simulink library "mylib"  (Simulink 9.2)
settings: Solver=VariableStepAuto  StartTime=0.0  StopTime=10.0  RelTol=1e-3
values from neighbouring files (symbols this model uses):
  FLINT32_MAX = flintmax('single')    [lib_consts.m]
undefined symbols (not defined in the file or in its folder): BAR_2_Pa, CC_2_M3, CCpREV_2_M3pRAD, DEG_2_RAD, DiscIntNeverNeededParam, G_2_MPS2, KNOTS_2_KPH, KPH_2_KNOTS, KPH_2_MPS, kXX_2_XX, M3_2_CC, M3pRAD_2_CCpREV, MPS2_2_G, MPS_2_KPH, Pa_2_BAR, RAD_2_DEG, RADpS_2_RPM, RPM_2_RADpS, XX_2_kXX
libraries: $bdroot x12, simulink x4, Ricardo_SW_dev_lib x1
(part 2 of 2)

== system mylib/Universals/Subsystem ==
  In1 : Inport
      settings: AttributesFormatString=<tsample=%<SampleTime>>
  Out1 : Outport
      settings: AttributesFormatString=<tsample=%<SampleTime>>
  wires:
  In1/1 -> Out1/1

== system mylib/Universals/Switch Case Action Subsystem ==
  In1 : Inport
      settings: AttributesFormatString=<tsample=%<SampleTime>>
  Action Port : ActionPort  ActionType=case
  Out1 : Outport
      settings: AttributesFormatString=<tsample=%<SampleTime>>
  wires:
  In1/1 -> Out1/1

== system mylib/Universals/Variant Subsystem ==
  note: 1) Only subsystems can be added as variant choices at this level
      | 2) Blocks cannot be connected at this level as connectivity is
      | automatically determined at simulation, based on the active variant
  In1 : Inport
      settings: AttributesFormatString=<tsample=%<SampleTime>>
  Out1 : Outport
      settings: AttributesFormatString=<tsample=%<SampleTime>>

== system mylib/Counter&Timer/Counter_Up/Delay_IV ==
  u : Inport
  IV : Inport  Port=2
  Constant4 : Constant  Value=0
  Data Type Conversion4 : DataTypeConversion
  Switch : Switch  Criteria=u2 ~= 0  Threshold=0.5  RndMeth=Zero
      settings: AttributesFormatString=<threshold=%<threshold>>\n<criteria=%<Criteria>>
  Unit Delay : UnitDelay  InitialCondition=1  SampleTime=-1
      settings: AttributesFormatString=<initial=%<x0>>\n<tsample=%<sampleTime>>
  Unit Delay1 : UnitDelay  SampleTime=-1
      settings: AttributesFormatString=<initial=%<x0>>\n<tsample=%<sampleTime>>
  y : Outport
  wires:
  Data Type Conversion4/1 -> Unit Delay/1
  Constant4/1 -> Data Type Conversion4/1
  IV/1 -> Switch/1
  u/1 -> Unit Delay1/1
  Switch/1 -> y/1
  Unit Delay/1 -> Switch/2
  Unit Delay1/1 -> Switch/3

== system mylib/Counter&Timer/rolling_edge_counter/boolean_edge ==
  note: Detect false to true boolean edge
  input_flg : Inport
      settings: AttributesFormatString=<tsample=%<SampleTime>>
  Logical Operator1 : Logic  AllPortsSameDT=off  OutDataTypeStr=boolean
  Logical Operator2 : Logic  Operator=NOT  AllPortsSameDT=off  OutDataTypeStr=boolean
  Unit Delay : UnitDelay  InitialCondition=false  SampleTime=-1
      settings: AttributesFormatString=<initial=%<x0>>\n<tsample=%<sampleTime>>
  edgle_flg : Outport
      settings: AttributesFormatString=<tsample=%<SampleTime>>
  wires:
  Unit Delay/1 -> Logical Operator2/1
  Logical Operator2/1 -> Logical Operator1/2
  Logical Operator1/1 -> edgle_flg/1  "edgle_flg"
  input_flg/1 -> Unit Delay/1, Logical Operator1/1  "input_flg"

== system mylib/Counter&Timer/rolling_edge_counter/conditional_counter ==
  note: Increment a rolling counter each time an edge is detected
  increment_on : Inport
      settings: AttributesFormatString=<tsample=%<SampleTime>>
  Constant : Constant  OutDataTypeStr=uint8  SampleTime=-1
      settings: AttributesFormatString=<tsample=%<SampleTime>>
  Sum : Sum  AccumDataTypeStr=uint8  RndMeth=Zero
  Switch : Switch  Criteria=u2 ~= 0  Threshold=0.5  RndMeth=Zero
      settings: AttributesFormatString=<threshold=%<threshold>>\n<criteria=%<Criteria>>
  Unit Delay1 : UnitDelay  SampleTime=-1
      settings: AttributesFormatString=<initial=%<x0>>\n<tsample=%<sampleTime>>
  rolling_ctr : Outport
      settings: AttributesFormatString=<tsample=%<SampleTime>>
  wires:
  increment_on/1 -> Switch/2  "increment_on"
  Constant/1 -> Sum/1
  Unit Delay1/1 -> Switch/3, Sum/2
  Sum/1 -> Switch/1
  Switch/1 -> Unit Delay1/1, rolling_ctr/1  "rolling_ctr"

== system mylib/PIDs/PI_FeedForward/clip_status ==
  max_dmd : Inport
      settings: AttributesFormatString=<tsample=%<SampleTime>>
  value : Inport  Port=2
      settings: AttributesFormatString=<tsample=%<SampleTime>>
  min_dmd : Inport  Port=3
      settings: AttributesFormatString=<tsample=%<SampleTime>>
  AboveMax : RelationalOperator  Operator=<  OutDataTypeStr=boolean  RndMeth=Nearest
  BelowMin : RelationalOperator  Operator=<  OutDataTypeStr=boolean  RndMeth=Nearest
  OutsideLimit : Logic  Operator=OR  AllPortsSameDT=off  OutDataTypeStr=boolean
  Switch : Switch  Criteria=u2 ~= 0  Threshold=0.5  RndMeth=Zero
      settings: AttributesFormatString=<threshold=%<threshold>>\n<criteria=%<Criteria>>
  Switch1 : Switch  Criteria=u2 ~= 0  Threshold=0.5  RndMeth=Zero
      settings: AttributesFormatString=<threshold=%<threshold>>\n<criteria=%<Criteria>>
  dmd : Outport
      settings: AttributesFormatString=<tsample=%<SampleTime>>
  off_limits : Outport  Port=2
      settings: AttributesFormatString=<tsample=%<SampleTime>>
  wires:
  OutsideLimit/1 -> off_limits/1
  max_dmd/1 -> Switch/1, AboveMax/1
  value/1 -> AboveMax/2, Switch1/3, BelowMin/1
  AboveMax/1 -> Switch/2, OutsideLimit/1
  Switch/1 -> dmd/1
  min_dmd/1 -> Switch1/1, BelowMin/2
  Switch1/1 -> Switch/3
  BelowMin/1 -> Switch1/2, OutsideLimit/2

== system mylib/PIDs/PI_FeedForward/deriv_term ==
  error : Inport
  Kd : Inport  Port=2
  deriv_Tc : Inport  Port=3
  dT : Inport  Port=4
  1st Order Filter : Ricardo_SW_dev_lib/1st Order Filter  SystemSampleTime=-1
  Product : Product  RndMeth=Zero
  Product1 : Product  Inputs=*/  RndMeth=Zero
  rawdmd : Sum  Inputs=+-  RndMeth=Zero
  d_term : Outport
      settings: AttributesFormatString=<tsample=%<SampleTime>>
  wires:
  error/1 -> rawdmd/1, 1st Order Filter/1
  Product/1 -> d_term/1  "d_term"
  Kd/1 -> Product/2
  deriv_Tc/1 -> Product1/2, 1st Order Filter/2
  dT/1 -> 1st Order Filter/3
  1st Order Filter/1 -> rawdmd/2
  rawdmd/1 -> Product1/1
  Product1/1 -> Product/1

== system mylib/PIDs/PI_FeedForward/integral_term ==
  error : Inport
  Ki : Inport  Port=2
  dT : Inport  Port=3
  i_reset : Inport  Port=4
  i_pause : Inport  Port=5
  Constant : Constant  Value=0  OutDataTypeStr=Inherit: Inherit via back propagation  SampleTime=-1
      settings: AttributesFormatString=<tsample=%<SampleTime>>
  Data Type Duplicate1 : DataTypeDuplicate  NumInputPorts=3
  Product2 : Product  Inputs=3  RndMeth=Zero
  Sum1 : Sum  RndMeth=Zero
  Switch : Switch  Criteria=u2 ~= 0  Threshold=0.5  RndMeth=Zero
      settings: AttributesFormatString=<threshold=%<threshold>>\n<criteria=%<Criteria>>
  Switch1 : Switch  Criteria=u2 ~= 0  Threshold=0.5  RndMeth=Zero
      settings: AttributesFormatString=<threshold=%<threshold>>\n<criteria=%<Criteria>>
  Unit Delay : UnitDelay  SampleTime=-1
      settings: AttributesFormatString=<initial=%<x0>>\n<tsample=%<sampleTime>>
  i_term : Outport
  wires:
  i_pause/1 -> Switch/2
  error/1 -> Data Type Duplicate1/1, Product2/1
  Ki/1 -> Product2/2
  Constant/1 -> Data Type Duplicate1/2, Switch1/1, Switch/1
  Product2/1 -> Switch/3
  Switch/1 -> Sum1/1
  Unit Delay/1 -> Data Type Duplicate1/3, Sum1/2
  Switch1/1 -> i_term/1, Unit Delay/1  "i_term"
  dT/1 -> Product2/3
  Sum1/1 -> Switch1/3
  i_reset/1 -> Switch1/2

== system mylib/PIDs/PI_FeedForward/prop_term ==
  Kp : Inport
  error : Inport  Port=2
  Product : Product  RndMeth=Zero
  p_term : Outport
      settings: AttributesFormatString=<tsample=%<SampleTime>>
  wires:
  Kp/1 -> Product/2
  Product/1 -> p_term/1  "p_term"
  error/1 -> Product/1

== system mylib/PIDs/PI_adjustable/clip_status ==
  max : Inport
      settings: AttributesFormatString=<tsample=%<SampleTime>>
  value : Inport  Port=2
      settings: AttributesFormatString=<tsample=%<SampleTime>>
  min : Inport  Port=3
      settings: AttributesFormatString=<tsample=%<SampleTime>>
  AboveMax : RelationalOperator  Operator=<  OutDataTypeStr=boolean  RndMeth=Nearest
  BelowMin : RelationalOperator  Operator=<  OutDataTypeStr=boolean  RndMeth=Nearest
  Switch : Switch  Criteria=u2 ~= 0  Threshold=0.5  RndMeth=Zero
      settings: AttributesFormatString=<threshold=%<threshold>>\n<criteria=%<Criteria>>
  Switch1 : Switch  Criteria=u2 ~= 0  Threshold=0.5  RndMeth=Zero
      settings: AttributesFormatString=<threshold=%<threshold>>\n<criteria=%<Criteria>>
  clipped_value : Outport
      settings: AttributesFormatString=<tsample=%<SampleTime>>
  above_max : Outport  Port=2
      settings: AttributesFormatString=<tsample=%<SampleTime>>
  below_min : Outport  Port=3
      settings: AttributesFormatString=<tsample=%<SampleTime>>
  wires:
  max/1 -> Switch/1, AboveMax/1
  value/1 -> AboveMax/2, Switch1/3, BelowMin/1
  AboveMax/1 -> Switch/2, above_max/1
  Switch/1 -> clipped_value/1
  min/1 -> Switch1/1, BelowMin/2
  Switch1/1 -> Switch/3
  BelowMin/1 -> below_min/1, Switch1/2

== system mylib/PIDs/PI_adjustable/integral_term ==
  Ki : Inport
  dT : Inport  Port=2
  obs_error : Inport  Port=3
  integral_pause : Inport  Port=4
  integral_reset : Inport  Port=5
  Constant : Constant  Value=0  OutDataTypeStr=Inherit: Inherit via back propagation  SampleTime=-1
      settings: AttributesFormatString=<tsample=%<SampleTime>>
  Data Type Duplicate1 : DataTypeDuplicate  NumInputPorts=3
  Product2 : Product  Inputs=3  RndMeth=Zero
  Sum1 : Sum  RndMeth=Zero
  Switch : Switch  Criteria=u2 ~= 0  Threshold=0.5  RndMeth=Zero
      settings: AttributesFormatString=<threshold=%<threshold>>\n<criteria=%<Criteria>>
  Switch1 : Switch  Criteria=u2 ~= 0  Threshold=0.5  RndMeth=Zero
      settings: AttributesFormatString=<threshold=%<threshold>>\n<criteria=%<Criteria>>
  Unit Delay : UnitDelay  SampleTime=-1
      settings: AttributesFormatString=<initial=%<x0>>\n<tsample=%<sampleTime>>
  integ_term : Outport
  wires:
  integral_pause/1 -> Switch/2
  obs_error/1 -> Data Type Duplicate1/1, Product2/1
  Ki/1 -> Product2/2
  Constant/1 -> Data Type Duplicate1/2, Switch1/1, Switch/1
  Product2/1 -> Switch/3
  Switch/1 -> Sum1/1
  Unit Delay/1 -> Data Type Duplicate1/3, Sum1/2
  Switch1/1 -> Unit Delay/1, integ_term/1
  dT/1 -> Product2/3
  Sum1/1 -> Switch1/3
  integral_reset/1 -> Switch1/2

== system mylib/PIDs/PI_adjustable/prop_term ==
  Kp : Inport
  obs_error : Inport  Port=2
  Product : Product  RndMeth=Zero
  prop_term : Outport
      settings: AttributesFormatString=<tsample=%<SampleTime>>
  wires:
  Kp/1 -> Product/2
  Product/1 -> prop_term/1
  obs_error/1 -> Product/1

== system mylib/Switchs/switch_ramp/switch_ramp ==
  u1 : Inport
  sw : Inport  Port=2
  u2 : Inport  Port=3
  up : Inport  Port=4
  lo : Inport  Port=5
  Chart : Stateflow chart  TreatAsAtomicUnit=on
  y : Outport
  RampOn : Outport  Port=2
  wires:
  Chart/2(RampOn) -> RampOn/1
  up/1 -> Chart/4(up)
  lo/1 -> Chart/5(lo)
  u2/1 -> Chart/3(u2)
  sw/1 -> Chart/2(swt)
  u1/1 -> Chart/1(u1)
  Chart/1(y) -> y/1

== system mylib/Universals/DocBlockDescription/EmptySubsystem ==

== system mylib/Universals/DocBlockHistory/EmptySubsystem ==

== stateflow chart Universals/Chart ==

== stateflow chart BitsMask/bitmask16/mask16 ==
  (default) -> (junction 10) : {
      | result=0;
      | nbit=0;
      | }
  (junction 10) -> (junction 11) [order 2]
  (junction 13) -> (junction 10)
  (junction 10) -> (junction 12) [order 1] : [ nbit < num_bits]
  (junction 12) -> (junction 13) : {
      |   masked_val = (data[nbit] << nbit);
      |   result = result | masked_val;
      |   nbit = nbit + 1;
      | }
  data: data input uint16; num_bits input uint8; masked_val local uint16; nbit local uint8; result output uint16

== stateflow chart BitsMask/bitmask32/mask32 ==
  (default) -> (junction 26) : {
      | result=0;
      | nbit=0;
      | }
  (junction 26) -> (junction 27) [order 2]
  (junction 29) -> (junction 26)
  (junction 26) -> (junction 28) [order 1] : [ nbit < num_bits]
  (junction 28) -> (junction 29) : {
      |   masked_val = (data[nbit] << nbit);
      |   result = result | masked_val;
      |   nbit = nbit + 1;
      | }
  data: data input uint32; num_bits input uint8; masked_val local uint32; nbit local uint8; result output uint32

== stateflow chart BitsMask/bitmask8/mask8 ==
  (default) -> (junction 42) : {
      | result=0;
      | nbit=0;
      | }
  (junction 42) -> (junction 43) [order 2]
  (junction 45) -> (junction 42)
  (junction 42) -> (junction 44) [order 1] : [ nbit < num_bits]
  (junction 44) -> (junction 45) : {
      |   masked_val = (data[nbit] << nbit);
      |   result = result | masked_val;
      |   nbit = nbit + 1;
      | }
  data: data input uint8; num_bits input uint8; masked_val local uint8; nbit local uint8; result output uint8

== stateflow chart Delay/debounce/timed_debounce ==
  state OFF
    (default) -> (junction 57)
    OFF -> (junction 57) [order 1]
    (junction 57) -> (junction 58) : {flg_out = false;}
  state ON_WAIT
    (default) -> (junction 62) : {t_wait = 0;}
    ON_WAIT -> (junction 62) [order 1]
    (junction 62) -> (junction 63) : {
        | t_wait += t_step;
        | flg_out = false;
        | }
  state ON
    (default) -> (junction 67)
    ON -> (junction 67) [order 1]
    (junction 67) -> (junction 68) : {flg_out = true;}
  state OFF_WAIT
    (default) -> (junction 72) : {t_wait = 0;}
    OFF_WAIT -> (junction 72) [order 1]
    (junction 72) -> (junction 73) : {
        | t_wait += t_step;
        | flg_out = true;
        | }
  (default) -> (junction 83)
  (junction 83) -> (junction 84) [order 1] : [flg_in]
  (junction 83) -> OFF [order 2]
  (junction 84) -> ON
  OFF -> (junction 85) [order 1] : [flg_in]
  (junction 85) -> ON [order 1] : [t_delay_on == 0]
  (junction 85) -> ON_WAIT [order 2]
  ON_WAIT -> ON [order 2] : [t_wait > t_delay_on - t_step]
  ON_WAIT -> OFF [order 1] : [!flg_in]
  ON -> (junction 86) [order 1] : [!flg_in]
  (junction 86) -> OFF [order 1] : [t_delay_off == 0]
  (junction 86) -> OFF_WAIT [order 2]
  OFF_WAIT -> OFF [order 2] : [t_wait > t_delay_off - t_step]
  OFF_WAIT -> ON [order 1] : [flg_in]
  data: flg_in input boolean; t_delay_on input single; t_delay_off input single; t_step input single; flg_out output boolean; t_wait local single

== stateflow chart Switchs/switch_ramp/switch_ramp/Chart ==
  state U2_TO_U1
    state U2_TO_U1_INC
      en:
      RampOn = true;
      err = u1 - y;
      y = min(max(y + min(err, up), u2), u1);
      du:
      err = u1 - y;
      y = min(max(y + min(err, up), u2), u1);
    state U2_TO_U1_DEC
      en:
      RampOn = true;
      err = u1 - y;
      y = max(min(y + max(err, lo), u2), u1);
      du:
      err = u1 - y;
      y = max(min(y + max(err, lo), u2), u1);
  state U2
    en:
    RampOn = false;
    y = u2;
    du:
    y = u2;
  state U1
    en:
    RampOn = false;
    y = u1;
    du:
    y = u1;
  state U1_TO_U2
    state U1_TO_U2_INC
      en:
      RampOn = true;
      err = u2 - y;
      y = min(max(y + min(err, up), u1), u2);
      du:
      err = u2 - y;
      y = min(max(y + min(err, up), u1), u2);
    state U1_TO_U2_DEC
      en:
      RampOn = true;
      err = u2 - y;
      y = max(min(y + max(err, lo), u1), u2);
      du:
      err = u2 - y;
      y = max(min(y + max(err, lo), u1), u2);
  (default) -> U2
  (junction 119) -> U2_TO_U1_INC [order 1] : [u1 >= u2]
  U2_TO_U1_INC -> U1 : [(u1 - y) <= up]
  U2 -> (junction 119) : [swt == 1]
  (junction 119) -> U2_TO_U1_DEC [order 2]
  U2_TO_U1_DEC -> U1 : [(u1 - y) >= lo]
  U1_TO_U2 -> (junction 119) : [swt == 1]
  U2_TO_U1 -> (junction 120) : [swt == 0]
  U1_TO_U2_INC -> U2 : [(u2 - y) <= up]
  (junction 120) -> U1_TO_U2_INC [order 1] : [u2 >= u1]
  U1 -> (junction 120) : [swt == 0]
  (junction 120) -> U1_TO_U2_DEC [order 2]
  U1_TO_U2_DEC -> U2 : [(u2 - y) >= lo]
  data: y output single; u1 input single; swt input boolean; RampOn output boolean; u2 input single; err local single; up input single; lo input single

== stateflow chart Delay/turnOFF_delay/timed_delay ==
  state OFF
    (default) -> (junction 139)
    OFF -> (junction 139) [order 1]
    (junction 139) -> (junction 140) : {flg_out = false;}
  state OFF_WAIT
    (default) -> (junction 144) : {t_wait = 0;}
    OFF_WAIT -> (junction 144) [order 1]
    (junction 144) -> (junction 145) : {
        | t_wait += t_step;
        | flg_out = true;
        | }
  state ON
    (default) -> (junction 149)
    ON -> (junction 149) [order 1]
    (junction 149) -> (junction 150) : {flg_out = true;}
  (default) -> (junction 159)
  (junction 159) -> (junction 160) [order 1] : [flg_in]
  (junction 159) -> OFF [order 2]
  (junction 160) -> ON
  OFF -> ON [order 1] : [flg_in]
  ON -> (junction 161) [order 1] : [!flg_in]
  (junction 161) -> OFF [order 1] : [t_delay_off == 0]
  (junction 161) -> OFF_WAIT [order 2]
  OFF_WAIT -> OFF [order 2] : [t_wait > t_delay_off - t_step]
  OFF_WAIT -> ON [order 1] : [flg_in]
  data: flg_in input boolean; t_delay_off input single; t_step input single; flg_out output boolean; t_wait local single

== stateflow chart Delay/turnON_delay/timed_delay ==
  state OFF
    (default) -> (junction 177)
    OFF -> (junction 177) [order 1]
    (junction 177) -> (junction 178) : {flg_out = false;}
  state ON_WAIT
    (default) -> (junction 182) : {t_wait = 0;}
    ON_WAIT -> (junction 182) [order 1]
    (junction 182) -> (junction 183) : {
        | t_wait += t_step;
        | flg_out = false;
        | }
  state ON
    (default) -> (junction 187)
    ON -> (junction 187) [order 1]
    (junction 187) -> (junction 188) : {flg_out = true;}
  (default) -> (junction 197)
  (junction 197) -> (junction 198) [order 1] : [flg_in]
  (junction 197) -> OFF [order 2]
  (junction 198) -> ON
  OFF -> (junction 199) [order 1] : [flg_in]
  (junction 199) -> ON [order 1] : [t_delay_on == 0]
  (junction 199) -> ON_WAIT [order 2]
  ON_WAIT -> ON [order 2] : [t_wait > t_delay_on-t_step]
  ON_WAIT -> OFF [order 1] : [!flg_in]
  ON -> OFF [order 1] : [!flg_in]
  data: flg_in input boolean; t_delay_on input single; t_step input single; flg_out output boolean; t_wait local single
